simulink model "doc_hamming_check"  (R2014a)
settings: Solver=VariableStepDiscrete  StartTime=0.0  StopTime=inf  RelTol=1e-3
undefined symbols (not defined in the file or in its folder): qfunc, randseed
libraries: commblkcod2 x3, commdigbbndpm3 x2, commchan3 x2, commsink2 x2, commrandsrc2 x1
settings Model: Creator=The MathWorks Inc.
settings DataIOCC: SignalLoggingSaveFormat=ModelDataLogs  SignalLoggingName=sigsOut
settings OptimizationCC: ExpressionDepthLimit=2147483647  InitFltsAndDblsToZero=on
settings DebuggingCC: SaveWithParameterizedLinksMsg=none  UnderspecifiedInitializationDetection=Classic  SignalResolutionControl=TryResolveAllWithWarning  SolverPrmCheckMsg=none  MultiTaskDSMMsg=warning  MultiTaskCondExecSysMsg=none  FcnCallInpInsideContextMsg=UseLocalSettings  StateNameClashWarn=warning  StrictBusMsg=None
settings HardwareCC: TargetUnknown=on
settings RTWCC: IncludeERTFirstTime=on
settings GRTTargetCC: TargetFcnLib=ansi_tfl_tmw.mat  CombineOutputUpdateFcns=off  GRTInterface=on

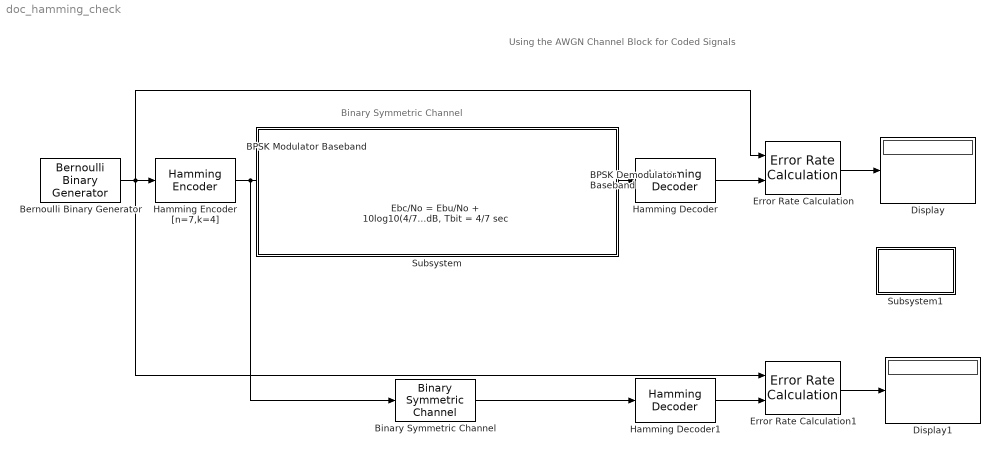
== system doc_hamming_check ==
  note: Binary Symmetric Channel
  note: Using the AWGN Channel Block for Coded Signals
  BPSK Demodulator Baseband : commdigbbndpm3/BPSK Demodulator Baseband  Ph=0  DecType=Hard decision  VarSource=Dialog  Variance=1  outDtype=double  derotateFactorWordLen=16
  BPSK Modulator Baseband : commdigbbndpm3/BPSK Modulator Baseband  Ph=0  outDtype=double  outWordLen=16  outUDDataType=sfix(16)  outFracLenMode=Best precision  outFracLen=15
  Bernoulli Binary Generator : commrandsrc2/Bernoulli Binary Generator  P=0.5  seed=randseed(61)  Ts=1  frameBased=on  sampPerFrame=4  orient=off  outDataType=double
  Binary Symmetric Channel : commchan3/Binary Symmetric Channel  P=qfunc(sqrt(2*10.^((8 + 10*log10(4/7))/10)))  s=67  E=off  outDtype=double
  Display : Display
  Display1 : Display
  "Ebc/No = Ebu/No + 10log10(4/7) dB, Tbit = 4/7 sec" : commchan3/AWGN Channel  InputProcessing=Columns as channels (frame based)  seed=67  noiseMode="Signal to noise ratio  (Eb/No)"  EbNodB=8 + 10*log10(4/7)  EsNodB=6.75 + 10*log10(4/7)  SNRdB=10  bitsPerSym=1  Ps=1  Tsym=4/7  variance=1
  Error Rate Calculation : commsink2/Error Rate Calculation  N=0  st_delay=0  cp_mode=Entire frame  subframe=[]  PMode=Port  WsName=ErrorVec  RsMode2=off  stop=on  numErr=200  maxBits=1e6
  Error Rate Calculation1 : commsink2/Error Rate Calculation  N=0  st_delay=0  cp_mode=Entire frame  subframe=[]  PMode=Port  WsName=ErrorVec  RsMode2=off  stop=on  numErr=200  maxBits=1e6
  Hamming Decoder : commblkcod2/Hamming Decoder  n=7  k=4
  Hamming Decoder1 : commblkcod2/Hamming Decoder  n=7  k=4
  Hamming Encoder [n=7,k=4] : commblkcod2/Hamming Encoder  n=7  k=4
  Subsystem : Subsystem
      mask Display: disp('')
  Subsystem1 : Subsystem
      mask Display: disp('Info')
  wires:
  BPSK Modulator Baseband/1 -> "Ebc/No = Ebu/No + 10log10(4/7) dB, Tbit = 4/7 sec"/1
  "Ebc/No = Ebu/No + 10log10(4/7) dB, Tbit = 4/7 sec"/1 -> BPSK Demodulator Baseband/1
  Error Rate Calculation/1 -> Display/1
  Bernoulli Binary Generator/1 -> Hamming Encoder [n=7,k=4]/1, Error Rate Calculation/1, Error Rate Calculation1/1
  Hamming Encoder [n=7,k=4]/1 -> Binary Symmetric Channel/1, BPSK Modulator Baseband/1
  BPSK Demodulator Baseband/1 -> Hamming Decoder/1
  Hamming Decoder/1 -> Error Rate Calculation/2
  Binary Symmetric Channel/1 -> Hamming Decoder1/1
  Hamming Decoder1/1 -> Error Rate Calculation1/2
  Error Rate Calculation1/1 -> Display1/1

== system doc_hamming_check/Subsystem ==

== system doc_hamming_check/Subsystem1 ==
  note: This example shows the usage of the AWGN Channel block for a signal with error control coding.
      | Both links are set for an uncoded Eb/No of 8 dB.  In the top link, the AWGN channel block is set to
      | provide a coded Eb/No of 8 + 10log10(4/7) dB, where 4/7 is the code rate.  This accounts for the fact
      | that the coded Eb/No is always lower (by a factor of the code rate) than the uncoded Eb/No.  The blue
      | shaded portion of the top link is simply a binary symmetric channel, which is modeled more
      | compactly in the bottom link.  The channel error probability of the top link is Q(sqrt(2*Ebc/No)),
      | where Q() is the standard Q function and Ebc/No is the coded Eb/No (in absolute terms, not in dB).
      |
      | For this example, it is important to note that the bit period at the input of the AWGN Channel block
      | is 4/7 sec.  It is 1 sec at the input of the Hamming Encoder block, but that block decreases the bit
      | time by a factor of the code rate.
      |
      | If you allow the model to run for 1e6 bits, you'll note that the BERs are virtually identical.  The
      | difference lies in the stochastic nature of the two random number generators.
      |
      | You can also check these BER results against expected analytical results by typing
      |
      | BER = bercoding(8, 'block', 'hard', 7, 4, 3)
      |
      | at the MATLAB command prompt.  This expression finds the upper bound of the BER of a linear,
      | rate 4/7 block code with a minimum distance of 3, and hard decision decoding.
